simulink model "ropod_KinModTest"  (R2016b)
settings: Solver=FixedStepAuto  StartTime=0.0  StopTime=timesim(end)  FixedStep=Ts  MaxStep=1e-3  RelTol=1e-3
values from neighbouring files (symbols this model uses):
  robot_par = [d_w s_w r_w CW_L]    [Ropod_kinematic_model_test.m]
  Ts = 1/200    (= 0.005)    [Ropod_kinematic_model_test.m]
undefined symbols (not defined in the file or in its folder): DiscIntNeverNeededParam
settings Model: Creator=cesar  LastModifiedBy=cesar

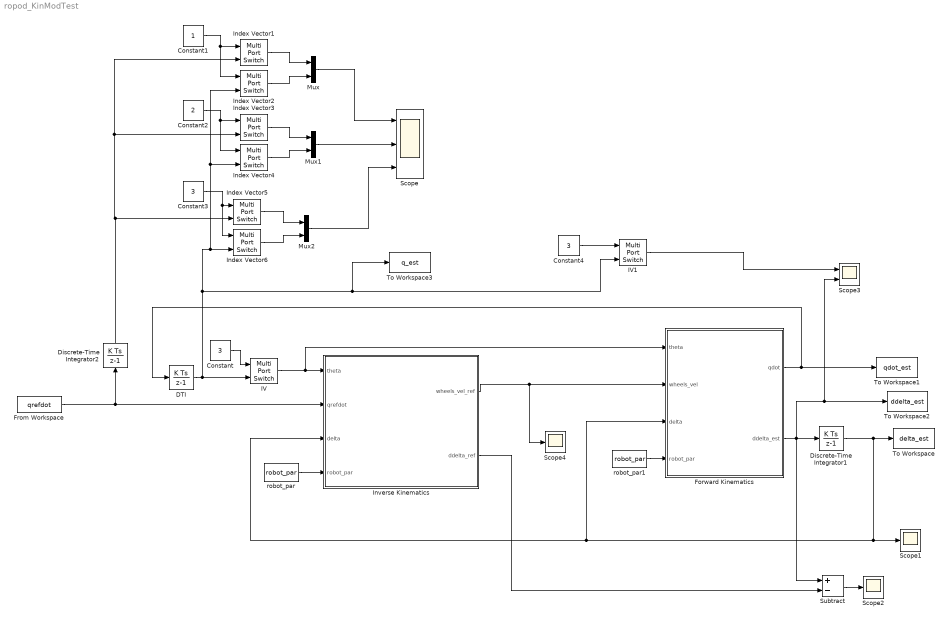
== system ropod_KinModTest ==
  Constant : Constant  Value=3
  Constant1 : Constant
  Constant2 : Constant  Value=2
  Constant3 : Constant  Value=3
  Constant4 : Constant  Value=3
  DTI : DiscreteIntegrator  InitialConditionSetting=State (most efficient)  SampleTime=Ts  ICPrevOutput=DiscIntNeverNeededParam  ICPrevScaledInput=DiscIntNeverNeededParam
  Discrete-Time Integrator1 : DiscreteIntegrator  InitialCondition=0*pi/2  InitialConditionSetting=State (most efficient)  SampleTime=Ts  ICPrevOutput=DiscIntNeverNeededParam  ICPrevScaledInput=DiscIntNeverNeededParam
  Discrete-Time Integrator2 : DiscreteIntegrator  InitialConditionSetting=State (most efficient)  SampleTime=Ts  ICPrevOutput=DiscIntNeverNeededParam  ICPrevScaledInput=DiscIntNeverNeededParam
  Forward Kinematics : MATLAB Function  TreatAsAtomicUnit=on
  From Workspace : FromWorkspace  VariableName=qrefdot  SampleTime=0
  IV : MultiPortSwitch  Inputs=1
  IV1 : MultiPortSwitch  Inputs=1
  Index Vector{1..6} (6 alike) : MultiPortSwitch  Inputs=1
  Inverse Kinematics : MATLAB Function  TreatAsAtomicUnit=on
  Mux : Mux  Inputs=2
  Mux1 : Mux  Inputs=2
  Mux2 : Mux  Inputs=2
  Scope : Scope  NumInputPorts=3
  Scope1 : Scope
  Scope2 : Scope
  Scope3 : Scope  NumInputPorts=2
  Scope4 : Scope
  Subtract : Sum  Inputs=+-
  To Workspace : ToWorkspace  VariableName=delta_est  SaveFormat=Timeseries  SampleTime=-1
  To Workspace1 : ToWorkspace  VariableName=qdot_est  SaveFormat=Timeseries  SampleTime=-1
  To Workspace2 : ToWorkspace  VariableName=ddelta_est  SaveFormat=Timeseries  SampleTime=-1
  To Workspace3 : ToWorkspace  VariableName=q_est  SaveFormat=Timeseries  SampleTime=-1
  robot_par : Constant  Value=robot_par
  robot_par1 : Constant  Value=robot_par
  wires:
  Constant/1 -> IV/1
  IV/1 -> Inverse Kinematics/1(theta), Forward Kinematics/1(theta)
  Inverse Kinematics/1(wheels_vel_ref) -> Scope4/1, Forward Kinematics/2(wheels_vel)
  Mux/1 -> Scope/1
  Constant1/1 -> Index Vector2/1, Index Vector1/1
  Index Vector1/1 -> Mux/1
  Index Vector2/1 -> Mux/2
  Mux1/1 -> Scope/2
  Constant2/1 -> Index Vector3/1, Index Vector4/1
  Index Vector3/1 -> Mux1/1
  Index Vector4/1 -> Mux1/2
  Forward Kinematics/1(qdot) -> To Workspace1/1, DTI/1
  Mux2/1 -> Scope/3
  Index Vector5/1 -> Mux2/1
  Index Vector6/1 -> Mux2/2
  Constant3/1 -> Index Vector6/1, Index Vector5/1
  Forward Kinematics/2(ddelta_est) -> Subtract/1, Scope3/2, To Workspace2/1, Discrete-Time Integrator1/1
  DTI/1 -> IV/2, To Workspace3/1, IV1/2, Index Vector6/2, Index Vector4/2, Index Vector2/2
  Discrete-Time Integrator2/1 -> Index Vector3/2, Index Vector1/2, Index Vector5/2
  From Workspace/1 -> Discrete-Time Integrator2/1, Inverse Kinematics/2(qrefdot)
  Discrete-Time Integrator1/1 -> To Workspace/1, Forward Kinematics/3(delta), Inverse Kinematics/3(delta), Scope1/1
  robot_par/1 -> Inverse Kinematics/4(robot_par)
  robot_par1/1 -> Forward Kinematics/4(robot_par)
  Subtract/1 -> Scope2/1
  Inverse Kinematics/2(ddelta_ref) -> Subtract/2
  Constant4/1 -> IV1/1
  IV1/1 -> Scope3/1

== matlab function ropod_KinModTest/Forward Kinematics ==
  data: theta input; wheels_vel input; qdot output; delta input; ddelta_est output; robot_par input
function [ qdot, ddelta_est ] = KinMod_ropod( theta, wheels_vel, delta, robot_par)
% KinMod_8wheelPlatform Summary of this function goes here
%   Detailed explanation goes here
%  Input:

%  theta 
%   contains the absolute orientation of teh robot
%  wheels_vel
%   velocities from the wheels in rad/sec. See documentation for wheel order
%  delta 
%   is the measured orientation vector of the wheels pair 
%   (using the x axis of teh robot as reference). Thus size 4.
%  robot_par
%   contains the parameters of the robot

% Output:
%  qdot
%   Vector of velocities in the interial frame [xdot ydot omegadot]
%  ddelta_est
%   estimated derivative of angle, used only for simulation purposes

d_w = robot_par(1);  % [m] Distance between two wheels in a pair of wheels
s_w = robot_par(2);  % [m] Caster offset
r_w = robot_par(3);  % [m] radius of the wheel
CW_L = robot_par(4); % [m] In this case all wheels are symmetrically distributed
% CW contains the positions of the smart wheels
CW= [CW_L  CW_L -CW_L -CW_L;
     CW_L -CW_L -CW_L CW_L];
Nwheels = size(CW,2); 

V_wh =  zeros(2,Nwheels);
vW_W =  zeros(2,Nwheels);
vR_W =  zeros(2,Nwheels);
ddelta_est = zeros(Nwheels,1);
vR_R = [0;0];
wR_R = 0;

for i=1:Nwheels   
    V_wh(1,i)    = r_w* wheels_vel(2*i-1);  % vectors of wheels velocities in m/s per SW (column)
    V_wh(2,i)    = r_w* wheels_vel(2*i);

    % From wheel's velocity to pivot point velocity vevtor
    vW_W(:,i) = [   1/2     1/2 ;  ...  % The velocity vector will only have x component (by definition delta=0 is x)
                   -s_w/d_w    s_w/d_w]* V_wh(:,i);
    ddelta_est(i) = [-1/d_w 1/d_w]* V_wh(:,i);
                
    % Rotation to obtain pivot velocity vector in robot coordinates
    vR_W(:,i) = [   cos(delta(i))     -sin(delta(i)); ...
                    sin(delta(i))     cos(delta(i))]*vW_W(:,i);
               
    vR_R = vR_R +  1/Nwheels * vR_W(:,i);      
    wR_R = wR_R + 1/1/Nwheels/sum(CW(:,i).^2) * [-CW(2,i) CW(1,i)] * vR_W(:,i);
end        
ddelta_est = ddelta_est - wR_R;

% To convert to Inertial frame, velocities in robot coordinates need to be
% rotated by theta
vI_R = [   cos(theta)     -sin(theta); ...
                    sin(theta)     cos(theta)]*vR_R;
wI_R = wR_R;
    
qdot = [vI_R; wI_R];


end

== matlab function ropod_KinModTest/Inverse Kinematics ==
  data: theta input; qrefdot input; delta input; wheels_vel_ref output; robot_par input; ddelta_ref output
function [wheels_vel_ref,ddelta_ref]  = InvKinMod_ropod( theta, qrefdot, delta, robot_par)
%InvKinMod_8wheelPlatform 
% With the inverse kinematics, one can determine the needed wheel
% velocities for certain reference in the inertial frame. 

%  Input:
%  theta 
%   contains the absolute orientation of the robot
%  qrefdot 
%   contains the reference velocity vector in the inertial frame
%  delta
%   contains the orientation of each pair of wheels in the robot frame
%  robot_par
%   contains the parameters of the robot

%  Output:
%  wheels_vel_ref
%   velocities from the wheels in rad/sec. See documentation for wheel order


d_w = robot_par(1);  % [m] Distance between two wheels in a pair of wheels
s_w = robot_par(2);  % [m] Caster offset
r_w = robot_par(3);  % [m] radius of the wheel
CW_L = robot_par(4); % [m] In this case all wheels are symmetrically distributed
% CW contains the positions of the smart wheels
CW= [CW_L  CW_L -CW_L -CW_L;    
     CW_L -CW_L -CW_L CW_L];
Nwheels = size(CW,2); 



% Next step is to compute the ddelta_ref:

wheels_vel_ref = zeros(2*Nwheels,1);
ddelta_ref= zeros(Nwheels,1);
vR_W = zeros(2,Nwheels);
vW_W = zeros(2,Nwheels);
V_wh = zeros(2,Nwheels);


vI_R = [qrefdot(1); qrefdot(2)];
wI_R = qrefdot(3);

% To convert from Inertial frame, to Robot frame, velocities in inertia frame
% need to be rotated by - theta
vR_R = [   cos(-theta)     -sin(-theta); ...
    sin(-theta)     cos(-theta)]*vI_R;
wR_R = wI_R;


for i=1:Nwheels
    
   
        
    % Now we express the wheel velocity vector in terms of the robot
    % coordinates
    vR_W(:,i) = [1 0 -CW(2,i);
                 0 1  CW(1,i)]*[vR_R; wR_R];    
             
    % Then we need to compute the orientation angle
    
       % Rotation to obtain pivot velocity vector in wheel coordinates
    vW_W(:,i) = [   cos(-delta(i))     -sin(-delta(i)); ...
                    sin(-delta(i))     cos(-delta(i))]*vR_W(:,i);    
    
    
    % From pivot's velocity to wheel's velocity vevtor
    V_wh(:,i) = [   1, -d_w/(2*s_w);  ...
                    1,  d_w/(2*s_w)]* vW_W(:,i);
                
    ddelta_ref(i) = ( V_wh(2,i) - V_wh(1,i) )/d_w - wR_R;
                
    wheels_vel_ref(2*i-1)   = V_wh(1,i)/r_w;
    wheels_vel_ref(2*i)     = V_wh(2,i)/r_w;

end
